simulink model "kalman_filter_example"  (R2022a)
settings: Solver=VariableStepAuto  StartTime=0.0  StopTime=500  FixedStep=1  RelTol=1e-3
model workspace (MAT data in the model file):
  A = 0.0012
  Cp = 500
  Tinf = 296
  a = 0.01
  epsilon = 0.9
  heat_flow_delay = 20
  m = 0.004
  room_temp = 23
  sig = 5.67e-08
  u = 10
undefined symbols (not defined in the file or in its folder): Discrete, Time
libraries: ctrlSharedLib x1, simulink_extras x1, simulink x1
settings Model: Creator=brian  LastModifiedBy=brian
settings SolverCC: AlgebraicLoopSolver=TrustRegion
settings DebuggingCC: UnconnectedInputMsg=warning  UnconnectedOutputMsg=warning  UnconnectedLineMsg=warning  SFMachineParentedDataDiag=warning
settings SFSimCC: CustomCodeUndefinedFunction=UseInterfaceOnly

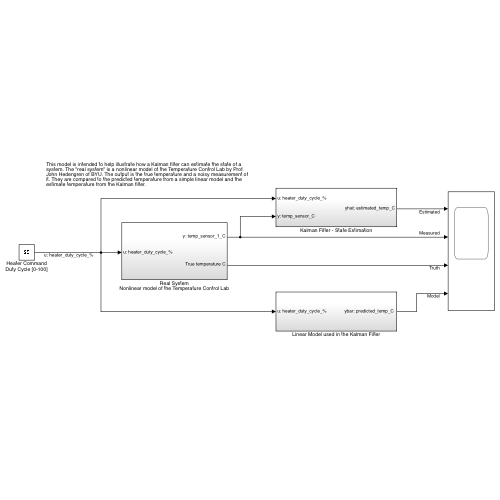
[thumbnail: Simulink's stored preview of the top-level diagram]
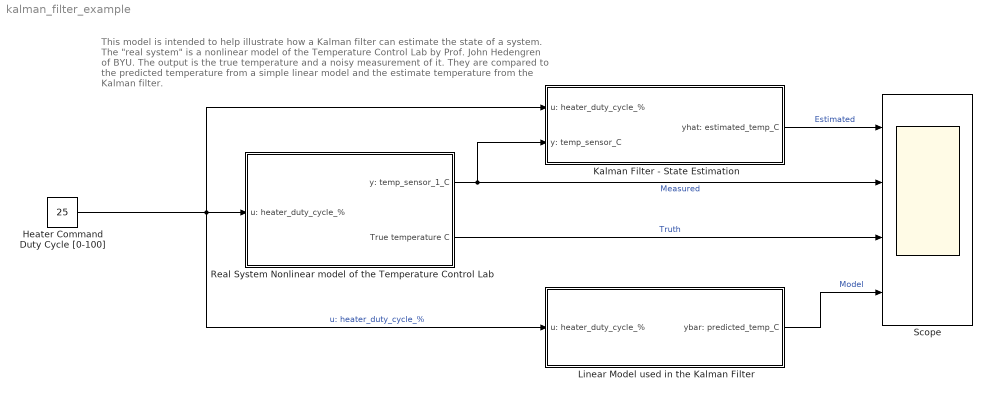
== system kalman_filter_example ==
  note: This model is intended to help illustrate how a Kalman filter can estimate the state of a system. The "real system" is a nonlinear model of the Temperature Control Lab by Prof. John Hedengren of BYU. The output is the true temperature and a noisy measurement of it. They are compared to the predicted temperature from a simple linear model and the estimate temperature from the Kalman filter.
  Heater Command Duty Cycle [0-100] : Constant  Value=25  SampleTime=-1
  Kalman Filter - State Estimation : Subsystem
  Linear Model used in the Kalman Filter : Subsystem
  Real System Nonlinear model of the Temperature Control Lab : Subsystem
  Scope : Scope  NumInputPorts=4
  wires:
  Real System Nonlinear model of the Temperature Control Lab/1(y: temp_sensor_1_C) -> Scope/2, Kalman Filter - State Estimation/2(y: temp_sensor_C)  "Measured"
  Heater Command Duty Cycle [0-100]/1 -> Linear Model used in the Kalman Filter/1(u: heater_duty_cycle_%), Kalman Filter - State Estimation/1(u: heater_duty_cycle_%), Real System Nonlinear model of the Temperature Control Lab/1(u: heater_duty_cycle_%)  "u: heater_duty_cycle_%"
  Real System Nonlinear model of the Temperature Control Lab/2(True temperature C) -> Scope/3  "Truth"
  Kalman Filter - State Estimation/1(yhat: estimated_temp_C) -> Scope/1  "Estimated"
  Linear Model used in the Kalman Filter/1("ybar: predicted_temp_C ") -> Scope/4  "Model"

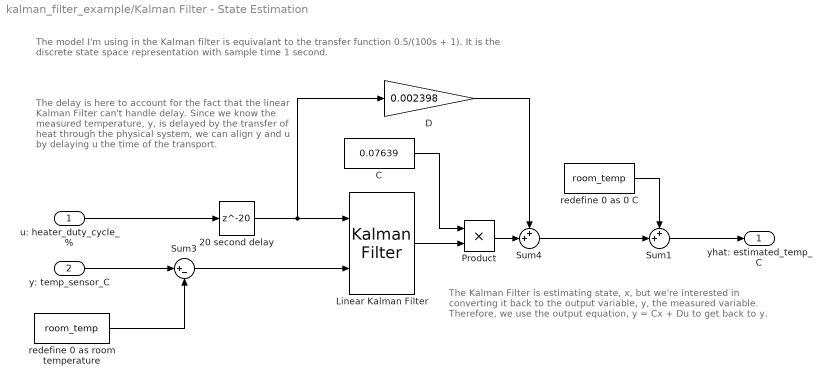
== system kalman_filter_example/Kalman Filter - State Estimation ==
  note: The model I'm using in the Kalman filter is equivalant to the transfer function 0.5/(100s + 1). It is the discrete state space representation with sample time 1 second.
  note: The delay is here to account for the fact that the linear Kalman Filter can't handle delay.
      |
      | Since we know the measured temperature, y, is delayed by the transfer of heat through the physical system, we can align y and u
      | by delaying u the time of the transport.
  note: The Kalman Filter is estimating state, x, but we're interested in converting it back to the output variable, y, the measured variable.
      | Therefore, we use the output equation, y = Cx + Du to get back to y.
  u: heater_duty_cycle_% : Inport
  y: temp_sensor_C : Inport  Port=2
  20 second delay : Delay  DelayLength=20  SampleTime=1
  C : Constant  Value=0.07639
  D : Gain  Gain=0.002398
  Linear Kalman Filter : ctrlSharedLib/Kalman Filter  TimeDomain=Discrete-Time  UseCurrentEstimator=on  ModelSource=Individual A, B, C, D matrices  ModelSourceVariable=ss(0.95,1,1,0,1)  A=0.991  B=0.0625  C=0.07639  D=0.002398  NumberOfStates=1  NumberOfInputs=1  NumberOfOutputs=1  InitialEstimateSource=Dialog  X0=0  P0=10  UseK=off  UseGH=off  NumberOfProcessNoiseInputs=1  G=1  TimeInvariantG=on  H=0  TimeInvariantH=on  Q=1  TimeInvariantQ=on  R=2  TimeInvariantR=on  N=0  TimeInvariantN=on  AddInputPort=on  AddEnablePort=off  OutputEstimatedY=off  OutputP=off  Ts=1
  Product : Product
  Sum1 : Sum  Inputs=++|
  Sum3 : Sum  Inputs=|+-
  Sum4 : Sum  Inputs=++|
  redefine 0 as 0 C : Constant  Value=room_temp
  redefine 0 as room temperature : Constant  Value=room_temp
  yhat: estimated_temp_C : Outport  VectorParamsAs1DForOutWhenUnconnected=off
  wires:
  Product/1 -> Sum4/2
  Linear Kalman Filter/1 -> Product/2
  redefine 0 as 0 C/1 -> Sum1/1
  Sum1/1 -> yhat: estimated_temp_C/1
  20 second delay/1 -> D/1, Linear Kalman Filter/1
  D/1 -> Sum4/1
  Sum4/1 -> Sum1/2
  u: heater_duty_cycle_%/1 -> 20 second delay/1
  Sum3/1 -> Linear Kalman Filter/2
  C/1 -> Product/1
  y: temp_sensor_C/1 -> Sum3/1
  redefine 0 as room temperature/1 -> Sum3/2

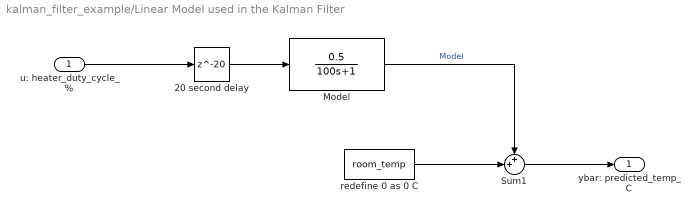
== system kalman_filter_example/Linear Model used in the Kalman Filter ==
  u: heater_duty_cycle_% : Inport
  20 second delay : Delay  DelayLength=20  SampleTime=1
  Model : TransferFcn  Numerator=0.5  Denominator=[100 1]
  Sum1 : Sum  Inputs=++|
  redefine 0 as 0 C : Constant  Value=room_temp
  "ybar: predicted_temp_C " : Outport
  wires:
  Sum1/1 -> "ybar: predicted_temp_C "/1
  Model/1 -> Sum1/1  "Model"
  redefine 0 as 0 C/1 -> Sum1/2
  u: heater_duty_cycle_%/1 -> 20 second delay/1
  20 second delay/1 -> Model/1

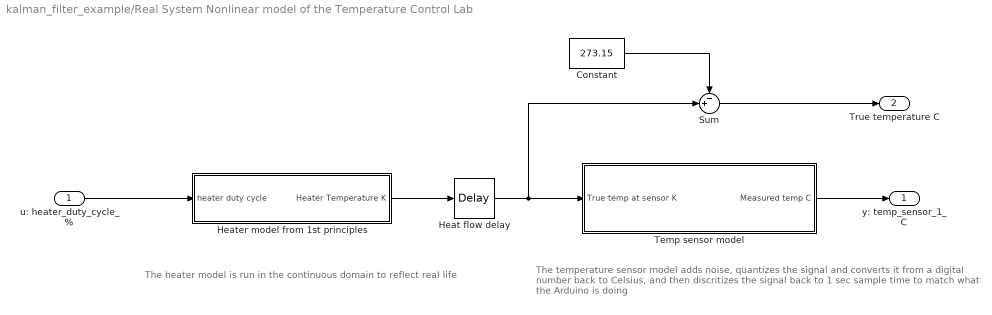
== system kalman_filter_example/Real System Nonlinear model of the Temperature Control Lab ==
  note: The heater model is run in the continuous domain to reflect real life
  note: The temperature sensor model adds noise, quantizes the signal and converts it from
      | a digital number back to Celsius, and then discritizes the signal back to 1 sec sample time
      | to match what the Arduino is doing
  u: heater_duty_cycle_% : Inport
  " Heater model from 1st principles" : Subsystem
  Constant : Constant  Value=273.15
  Heat flow delay : TransportDelay  DelayTime=heat_flow_delay  InitialOutput=Tinf
  Sum : Sum  Inputs=-+|
  Temp sensor model : Subsystem
  y: temp_sensor_1_C : Outport  VectorParamsAs1DForOutWhenUnconnected=off
  True temperature C : Outport  Port=2  VectorParamsAs1DForOutWhenUnconnected=off
  wires:
  u: heater_duty_cycle_%/1 -> " Heater model from 1st principles"/1(heater duty cycle)
  " Heater model from 1st principles"/1(Heater Temperature K) -> Heat flow delay/1
  Heat flow delay/1 -> Sum/2, Temp sensor model/1(True temp at sensor K)
  Temp sensor model/1(Measured temp C) -> y: temp_sensor_1_C/1
  Constant/1 -> Sum/1
  Sum/1 -> True temperature C/1

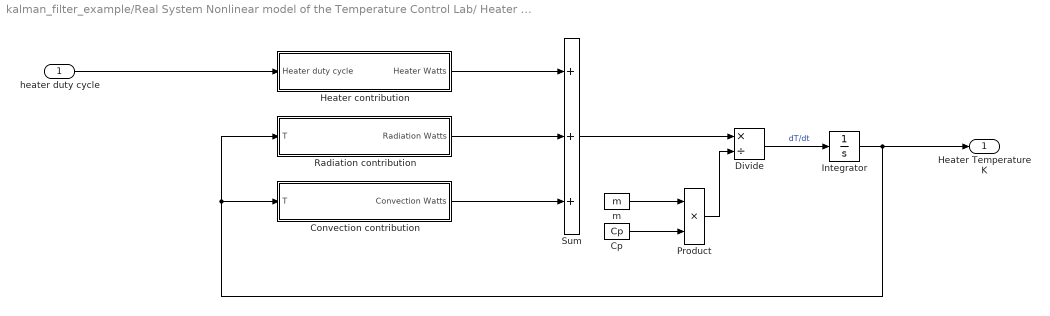
== system kalman_filter_example/Real System Nonlinear model of the Temperature Control Lab/ Heater model from 1st principles ==
  heater duty cycle : Inport
  Convection contribution : Subsystem
  Cp : Constant  Value=Cp
  Divide : Product  Inputs=*/
  Heater contribution : Subsystem
  Integrator : Integrator  InitialCondition=Tinf
  Product : Product
  Radiation contribution : Subsystem
  Sum : Sum  Inputs=+++
  m : Constant  Value=m
  Heater Temperature K : Outport  VectorParamsAs1DForOutWhenUnconnected=off
  wires:
  Divide/1 -> Integrator/1  "dT/dt"
  Cp/1 -> Product/2
  m/1 -> Product/1
  Sum/1 -> Divide/1
  Product/1 -> Divide/2
  Heater contribution/1(Heater Watts) -> Sum/1
  Radiation contribution/1(Radiation Watts) -> Sum/2
  Convection contribution/1(Convection Watts) -> Sum/3
  Integrator/1 -> Heater Temperature K/1, Convection contribution/1(T), Radiation contribution/1(T)
  heater duty cycle/1 -> Heater contribution/1(Heater duty cycle)

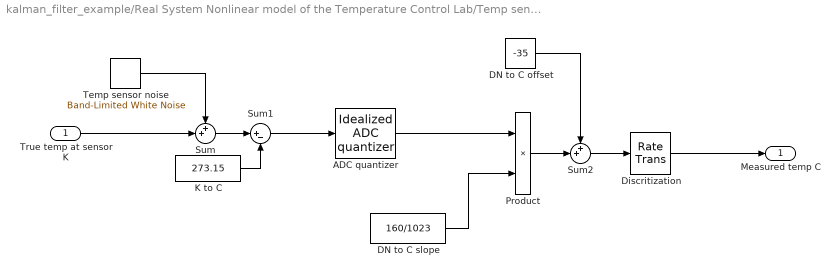
== system kalman_filter_example/Real System Nonlinear model of the Temperature Control Lab/Temp sensor model ==
  True temp at sensor K : Inport
  ADC quantizer : simulink_extras/Additional Discrete/Idealized ADC quantizer  NumberOfConverterBits=10  Vmin=-35  Vmax=125  OutputDataType=int16  OutputNegativeValues=off
  DN to C offset : Constant  Value=-35
  DN to C slope : Constant  Value=160/1023
  Discritization : RateTransition  InitialCondition=Tinf  OutPortSampleTime=1
  K to C : Constant  Value=273.15
  Product : Product
  Sum : Sum  Inputs=++|
  Sum1 : Sum  Inputs=|+-
  Sum2 : Sum  Inputs=++|
  Temp sensor noise : simulink/Sources/Band-Limited White Noise  Cov=0.06  Ts=1  seed=[23341]
  Measured temp C : Outport  VectorParamsAs1DForOutWhenUnconnected=off
  wires:
  Sum/1 -> Sum1/1
  Product/1 -> Sum2/2
  Discritization/1 -> Measured temp C/1
  DN to C offset/1 -> Sum2/1
  True temp at sensor K/1 -> Sum/2
  DN to C slope/1 -> Product/2
  Sum1/1 -> ADC quantizer/1
  Sum2/1 -> Discritization/1
  K to C/1 -> Sum1/2
  ADC quantizer/1 -> Product/1
  Temp sensor noise/1 -> Sum/1

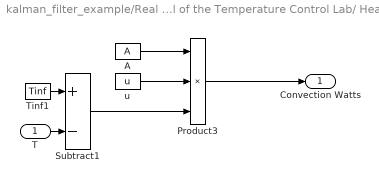
== system kalman_filter_example/Real System Nonlinear model of the Temperature Control Lab/ Heater model from 1st principles/Convection contribution ==
  T : Inport
  A : Constant  Value=A
  Product3 : Product  Inputs=3
  Subtract1 : Sum  Inputs=+-
  Tinf1 : Constant  Value=Tinf
  u : Constant  Value=u
  Convection Watts : Outport  VectorParamsAs1DForOutWhenUnconnected=off
  wires:
  A/1 -> Product3/1
  Tinf1/1 -> Subtract1/1
  T/1 -> Subtract1/2
  Subtract1/1 -> Product3/3
  u/1 -> Product3/2
  Product3/1 -> Convection Watts/1

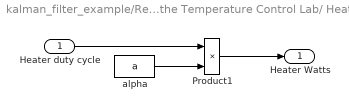
== system kalman_filter_example/Real System Nonlinear model of the Temperature Control Lab/ Heater model from 1st principles/Heater contribution ==
  Heater duty cycle : Inport
  Product1 : Product
  alpha : Constant  Value=a
  Heater Watts : Outport  VectorParamsAs1DForOutWhenUnconnected=off
  wires:
  Heater duty cycle/1 -> Product1/1
  Product1/1 -> Heater Watts/1
  alpha/1 -> Product1/2

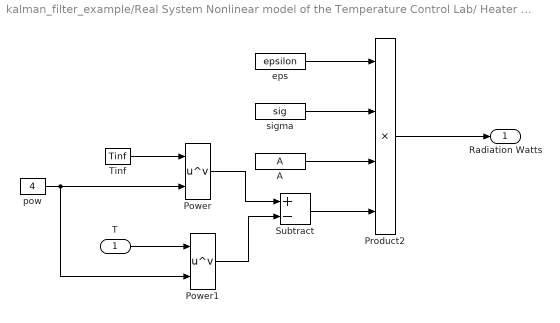
== system kalman_filter_example/Real System Nonlinear model of the Temperature Control Lab/ Heater model from 1st principles/Radiation contribution ==
  T : Inport
  A : Constant  Value=A
  Power : Math  Operator=pow  SignedPower=on
  Power1 : Math  Operator=pow  SignedPower=on
  Product2 : Product  Inputs=4
  Subtract : Sum  Inputs=+-
  Tinf : Constant  Value=Tinf
  eps : Constant  Value=epsilon
  pow : Constant  Value=4
  sigma : Constant  Value=sig
  Radiation Watts : Outport  VectorParamsAs1DForOutWhenUnconnected=off
  wires:
  Tinf/1 -> Power/1
  Power1/1 -> Subtract/2
  Product2/1 -> Radiation Watts/1
  Subtract/1 -> Product2/4
  T/1 -> Power1/1
  Power/1 -> Subtract/1
  sigma/1 -> Product2/2
  A/1 -> Product2/3
  eps/1 -> Product2/1
  pow/1 -> Power1/2, Power/2
